simulink subsystem "aeroParamsCalculation"  (R2025b)
settings: Solver=VariableStepAuto  StartTime=0.0  StopTime=10.0  RelTol=1e-3
values from neighbouring files (symbols this model uses):
  aeroParams : value not decoded    [plantParams.sldd]
libraries: simulink_extras x6, matrix_library x4
settings Model: Creator=maxhu  LastModifiedBy=maxhu

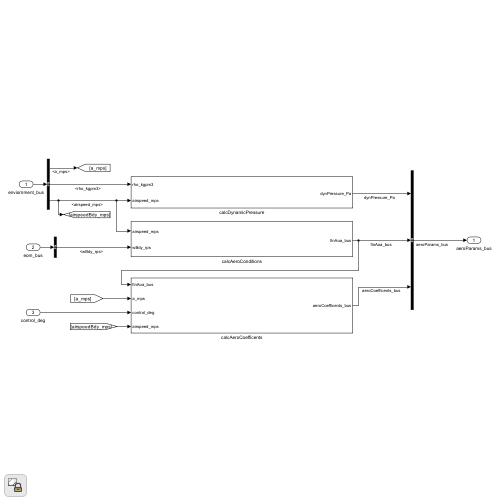
[thumbnail: Simulink's stored preview of the top-level diagram]
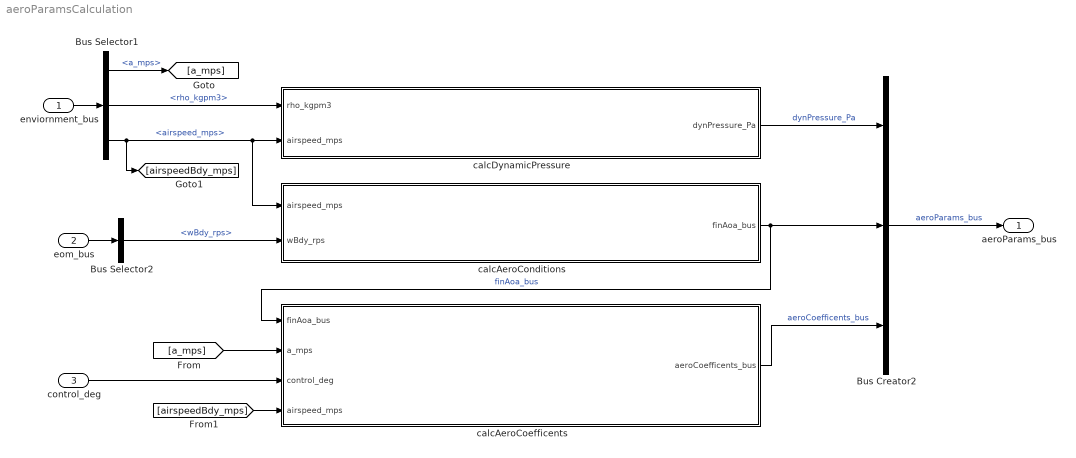
== system aeroParamsCalculation ==
  enviornment_bus : Inport
  eom_bus : Inport  Port=2
  control_deg : Inport  Port=3
  Bus Creator2 : BusCreator  Inputs=3
  Bus Selector1 : BusSelector  OutputSignals=a_mps,rho_kgpm3,airspeed_mps
  Bus Selector2 : BusSelector  OutputSignals=wBdy_rps
  calcAeroCoefficents : Subsystem
  calcAeroConditions : Subsystem
  calcDynamicPressure : Subsystem
  aeroParams_bus : Outport
  wires:
  enviornment_bus/1 -> Bus Selector1/1
  eom_bus/1 -> Bus Selector2/1
  Bus Creator2/1 -> aeroParams_bus/1  "aeroParams_bus"
  Bus Selector2/1 -> calcAeroConditions/2(wBdy_rps)  "<wBdy_rps>"
  Bus Selector1/2 -> calcDynamicPressure/1(rho_kgpm3)  "<rho_kgpm3>"
  calcAeroConditions/1(finAoa_bus) -> calcAeroCoefficents/1(finAoa_bus), Bus Creator2/2  "finAoa_bus"
  calcDynamicPressure/1(dynPressure_Pa) -> Bus Creator2/1  "dynPressure_Pa"
  Bus Selector1/1 -> [a_mps]  "<a_mps>"
  [a_mps] -> calcAeroCoefficents/2(a_mps)
  [airspeedBdy_mps] -> calcAeroCoefficents/4(airspeed_mps)
  control_deg/1 -> calcAeroCoefficents/3(control_deg)
  calcAeroCoefficents/1(aeroCoefficents_bus) -> Bus Creator2/3  "aeroCoefficents_bus"
  Bus Selector1/3 -> calcDynamicPressure/2(airspeed_mps), calcAeroConditions/1(airspeed_mps), [airspeedBdy_mps]  "<airspeed_mps>"

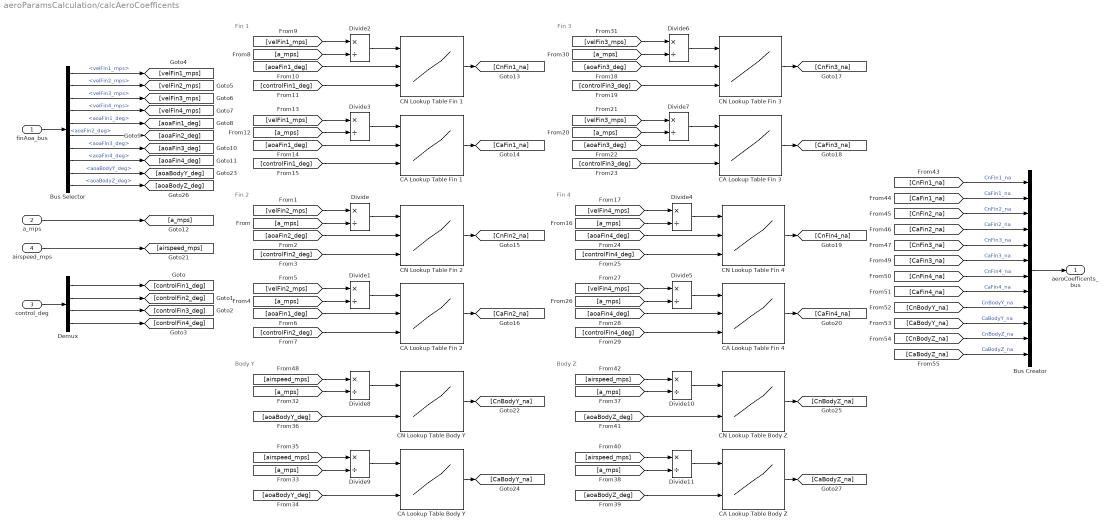
== system aeroParamsCalculation/calcAeroCoefficents ==
  note: Body Y
  note: Body Z
  note: Fin 4
  note: Fin 3
  note: Fin 1
  note: Fin 2
  finAoa_bus : Inport
  a_mps : Inport  Port=2
  control_deg : Inport  Port=3
  airspeed_mps : Inport  Port=4
  Bus Creator : BusCreator  Inputs=12
  Bus Selector : BusSelector  OutputSignals=velFin1_mps,velFin2_mps,velFin3_mps,velFin4_mps,aoaFin1_deg,aoaFin2_deg,aoaFin3_deg,aoaFin4_deg,aoaBodyY_deg,aoaBodyZ_deg
  CA Lookup Table Body Y : Lookup_n-D  BreakpointsForDimension1=aeroParams.machBreakpoints_na  BreakpointsForDimension2=aeroParams.aoaBreakpoints_deg  BreakpointsForDimension3=aeroParams.controlBreakpoints_deg  Table=aeroParams.CaBase_na  InternalRulePriority=Speed  RndMeth=Simplest
      settings: InputPortMap=u0,u1
  CA Lookup Table Body Z : Lookup_n-D  BreakpointsForDimension1=aeroParams.machBreakpoints_na  BreakpointsForDimension2=aeroParams.aoaBreakpoints_deg  BreakpointsForDimension3=aeroParams.controlBreakpoints_deg  Table=aeroParams.CaBase_na  InternalRulePriority=Speed  RndMeth=Simplest
      settings: InputPortMap=u0,u1
  CA Lookup Table Fin {1..4} (4 alike) : Lookup_n-D  NumberOfTableDimensions=3  BreakpointsForDimension1=aeroParams.machBreakpoints_na  BreakpointsForDimension2=aeroParams.aoaBreakpoints_deg  BreakpointsForDimension3=aeroParams.controlBreakpoints_deg  Table=aeroParams.CaFin_na  InternalRulePriority=Speed  RndMeth=Simplest
      settings: InputPortMap=u0,u1,u2
  CN Lookup Table Body Y : Lookup_n-D  BreakpointsForDimension1=aeroParams.machBreakpoints_na  BreakpointsForDimension2=aeroParams.aoaBreakpoints_deg  BreakpointsForDimension3=aeroParams.controlBreakpoints_deg  Table=aeroParams.CnBase_na  InternalRulePriority=Speed  RndMeth=Simplest
      settings: InputPortMap=u0,u1
  CN Lookup Table Body Z : Lookup_n-D  BreakpointsForDimension1=aeroParams.machBreakpoints_na  BreakpointsForDimension2=aeroParams.aoaBreakpoints_deg  BreakpointsForDimension3=aeroParams.controlBreakpoints_deg  Table=aeroParams.CnBase_na  InternalRulePriority=Speed  RndMeth=Simplest
      settings: InputPortMap=u0,u1
  CN Lookup Table Fin {1..4} (4 alike) : Lookup_n-D  NumberOfTableDimensions=3  BreakpointsForDimension1=aeroParams.machBreakpoints_na  BreakpointsForDimension2=aeroParams.aoaBreakpoints_deg  BreakpointsForDimension3=aeroParams.controlBreakpoints_deg  Table=aeroParams.CnFin_na  InternalRulePriority=Speed  RndMeth=Simplest
      settings: InputPortMap=u0,u1,u2
  Demux : Demux
  Divide{,1..11} (12 alike) : Product  Inputs=*/
  aeroCoefficents_bus : Outport
  wires:
  Bus Creator/1 -> aeroCoefficents_bus/1
  [CaBodyZ_na] -> Bus Creator/12  "CaBodyZ_na"
  [CnBodyZ_na] -> Bus Creator/11  "CnBodyZ_na"
  [CaBodyY_na] -> Bus Creator/10  "CaBodyY_na"
  [CnBodyY_na] -> Bus Creator/9  "CnBodyY_na"
  [CaFin4_na] -> Bus Creator/8  "CaFin4_na"
  [CnFin4_na] -> Bus Creator/7  "CnFin4_na"
  [CaFin3_na] -> Bus Creator/6  "CaFin3_na"
  [CnFin3_na] -> Bus Creator/5  "CnFin3_na"
  [CaFin2_na] -> Bus Creator/4  "CaFin2_na"
  [CnFin2_na] -> Bus Creator/3  "CnFin2_na"
  [CaFin1_na] -> Bus Creator/2  "CaFin1_na"
  [CnFin1_na] -> Bus Creator/1  "CnFin1_na"
  [a_mps] -> Divide10/2
  Divide10/1 -> CN Lookup Table Body Z/1
  [aoaBodyZ_deg] -> CN Lookup Table Body Z/2
  CN Lookup Table Body Z/1 -> [CnBodyZ_na]
  [aoaBodyZ_deg] -> CA Lookup Table Body Z/2
  CA Lookup Table Body Z/1 -> [CaBodyZ_na]
  [airspeed_mps] -> Divide11/1
  Divide11/1 -> CA Lookup Table Body Z/1
  [a_mps] -> Divide11/2
  [airspeed_mps] -> Divide10/1
  [airspeed_mps] -> Divide9/1
  [a_mps] -> Divide9/2
  Divide9/1 -> CA Lookup Table Body Y/1
  [aoaBodyY_deg] -> CA Lookup Table Body Y/2
  CA Lookup Table Body Y/1 -> [CaBodyY_na]
  Bus Selector/9 -> [aoaBodyY_deg]  "<aoaBodyY_deg>"
  Bus Selector/10 -> [aoaBodyZ_deg]  "<aoaBodyZ_deg>"
  [airspeed_mps] -> Divide8/1
  [aoaBodyY_deg] -> CN Lookup Table Body Y/2
  CN Lookup Table Body Y/1 -> [CnBodyY_na]
  [a_mps] -> Divide8/2
  Divide8/1 -> CN Lookup Table Body Y/1
  airspeed_mps/1 -> [airspeed_mps]
  CA Lookup Table Fin 4/1 -> [CaFin4_na]
  CN Lookup Table Fin 4/1 -> [CnFin4_na]
  CA Lookup Table Fin 3/1 -> [CaFin3_na]
  CN Lookup Table Fin 3/1 -> [CnFin3_na]
  CN Lookup Table Fin 2/1 -> [CnFin2_na]
  CA Lookup Table Fin 2/1 -> [CaFin2_na]
  CA Lookup Table Fin 1/1 -> [CaFin1_na]
  CN Lookup Table Fin 1/1 -> [CnFin1_na]
  Divide5/1 -> CA Lookup Table Fin 4/1
  [velFin4_mps] -> Divide4/1
  [aoaFin4_deg] -> CN Lookup Table Fin 4/2
  [controlFin4_deg] -> CN Lookup Table Fin 4/3
  [a_mps] -> Divide4/2
  [aoaFin3_deg] -> CN Lookup Table Fin 3/2
  [controlFin4_deg] -> CA Lookup Table Fin 4/3
  Divide6/1 -> CN Lookup Table Fin 3/1
  [aoaFin4_deg] -> CA Lookup Table Fin 4/2
  [a_mps] -> Divide5/2
  [velFin4_mps] -> Divide5/1
  Divide4/1 -> CN Lookup Table Fin 4/1
  [a_mps] -> Divide6/2
  [velFin3_mps] -> Divide7/1
  [aoaFin3_deg] -> CA Lookup Table Fin 3/2
  [controlFin3_deg] -> CA Lookup Table Fin 3/3
  [a_mps] -> Divide7/2
  [controlFin3_deg] -> CN Lookup Table Fin 3/3
  [velFin3_mps] -> Divide6/1
  Divide7/1 -> CA Lookup Table Fin 3/1
  Divide3/1 -> CA Lookup Table Fin 1/1
  [velFin1_mps] -> Divide2/1
  [aoaFin1_deg] -> CN Lookup Table Fin 1/2
  [controlFin1_deg] -> CN Lookup Table Fin 1/3
  [a_mps] -> Divide2/2
  [controlFin1_deg] -> CA Lookup Table Fin 1/3
  [aoaFin1_deg] -> CA Lookup Table Fin 1/2
  [a_mps] -> Divide3/2
  [velFin1_mps] -> Divide3/1
  Divide2/1 -> CN Lookup Table Fin 1/1
  [velFin2_mps] -> Divide1/1
  Divide1/1 -> CA Lookup Table Fin 2/1
  [controlFin2_deg] -> CA Lookup Table Fin 2/3
  [aoaFin1_deg] -> CA Lookup Table Fin 2/2
  [a_mps] -> Divide1/2
  [controlFin2_deg] -> CN Lookup Table Fin 2/3
  Bus Selector/8 -> [aoaFin4_deg]  "<aoaFin4_deg>"
  Bus Selector/7 -> [aoaFin3_deg]  "<aoaFin3_deg>"
  Bus Selector/6 -> [aoaFin2_deg]  "<aoaFin2_deg>"
  Bus Selector/5 -> [aoaFin1_deg]  "<aoaFin1_deg>"
  [aoaFin2_deg] -> CN Lookup Table Fin 2/2
  Divide/1 -> CN Lookup Table Fin 2/1
  [velFin2_mps] -> Divide/1
  [a_mps] -> Divide/2
  a_mps/1 -> [a_mps]
  Bus Selector/4 -> [velFin4_mps]  "<velFin4_mps>"
  Bus Selector/3 -> [velFin3_mps]  "<velFin3_mps>"
  Bus Selector/2 -> [velFin2_mps]  "<velFin2_mps>"
  Bus Selector/1 -> [velFin1_mps]  "<velFin1_mps>"
  finAoa_bus/1 -> Bus Selector/1
  Demux/4 -> [controlFin4_deg]
  Demux/3 -> [controlFin3_deg]
  Demux/2 -> [controlFin2_deg]
  Demux/1 -> [controlFin1_deg]
  control_deg/1 -> Demux/1

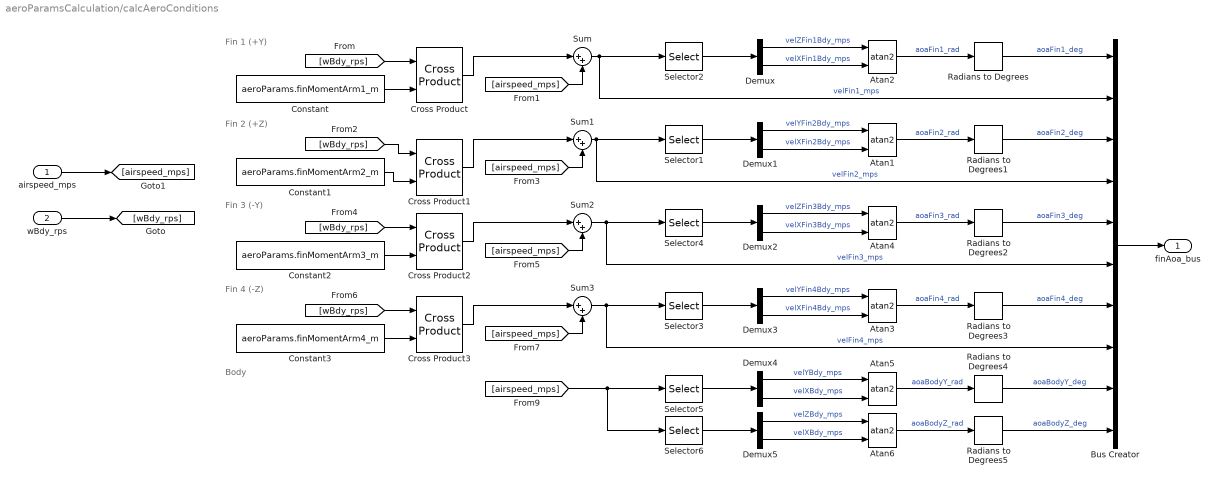
== system aeroParamsCalculation/calcAeroConditions ==
  note: Body
  note: Fin 1 (+Y)
  note: Fin 2 (+Z)
  note: Fin 3 (-Y)
  note: Fin 4 (-Z)
  airspeed_mps : Inport
  wBdy_rps : Inport  Port=2
  Atan{1..6} (6 alike) : Trigonometry  Operator=atan2
  Bus Creator : BusCreator  Inputs=10
  Constant : Constant  Value=aeroParams.finMomentArm1_m
  Constant1 : Constant  Value=aeroParams.finMomentArm2_m
  Constant2 : Constant  Value=aeroParams.finMomentArm3_m
  Constant3 : Constant  Value=aeroParams.finMomentArm4_m
  Cross Product{,1..3} (4 alike) : matrix_library/Cross Product
  Demux{,1..5} (6 alike) : Demux  Outputs=2
  Radians to Degrees{,1..5} (6 alike) : simulink_extras/Transformations/Radians to Degrees
  Selector1 : Selector  InputPortWidth=3  IndexOptions=Index vector (dialog)  Indices=[2 1]  OutputSizes=1
  Selector2 : Selector  InputPortWidth=3  IndexOptions=Index vector (dialog)  Indices=[3 1]  OutputSizes=1
  Selector3 : Selector  InputPortWidth=3  IndexOptions=Index vector (dialog)  Indices=[2 1]  OutputSizes=1
  Selector4 : Selector  InputPortWidth=3  IndexOptions=Index vector (dialog)  Indices=[3 1]  OutputSizes=1
  Selector5 : Selector  InputPortWidth=3  IndexOptions=Index vector (dialog)  Indices=[3 1]  OutputSizes=1
  Selector6 : Selector  InputPortWidth=3  IndexOptions=Index vector (dialog)  Indices=[2 1]  OutputSizes=1
  Sum{,1..3} (4 alike) : Sum  Inputs=|++
  finAoa_bus : Outport
  wires:
  Radians to Degrees5/1 -> Bus Creator/10  "aoaBodyZ_deg"
  Radians to Degrees4/1 -> Bus Creator/9  "aoaBodyY_deg"
  Selector6/1 -> Demux5/1
  Demux5/1 -> Atan6/1  "velZBdy_mps"
  Demux5/2 -> Atan6/2  "velXBdy_mps"
  Atan6/1 -> Radians to Degrees5/1  "aoaBodyZ_rad"
  Selector5/1 -> Demux4/1
  Atan5/1 -> Radians to Degrees4/1  "aoaBodyY_rad"
  Demux4/2 -> Atan5/2  "velXBdy_mps"
  [airspeed_mps] -> Selector6/1, Selector5/1
  Demux4/1 -> Atan5/1  "velYBdy_mps"
  Radians to Degrees3/1 -> Bus Creator/7  "aoaFin4_deg"
  Radians to Degrees2/1 -> Bus Creator/5  "aoaFin3_deg"
  Radians to Degrees1/1 -> Bus Creator/3  "aoaFin2_deg"
  Radians to Degrees/1 -> Bus Creator/1  "aoaFin1_deg"
  Bus Creator/1 -> finAoa_bus/1
  Atan3/1 -> Radians to Degrees3/1  "aoaFin4_rad"
  Atan4/1 -> Radians to Degrees2/1  "aoaFin3_rad"
  Atan1/1 -> Radians to Degrees1/1  "aoaFin2_rad"
  Atan2/1 -> Radians to Degrees/1  "aoaFin1_rad"
  Demux2/1 -> Atan4/1  "velZFin3Bdy_mps"
  Constant2/1 -> Cross Product2/2
  [airspeed_mps] -> Sum2/2
  Selector4/1 -> Demux2/1
  Cross Product2/1 -> Sum2/1
  [wBdy_rps] -> Cross Product2/1
  Sum3/1 -> Selector3/1, Bus Creator/8  "velFin4_mps"
  [wBdy_rps] -> Cross Product3/1
  [airspeed_mps] -> Sum3/2
  Constant3/1 -> Cross Product3/2
  Cross Product3/1 -> Sum3/1
  Selector3/1 -> Demux3/1
  Demux3/1 -> Atan3/1  "velYFin4Bdy_mps"
  Demux3/2 -> Atan3/2  "velXFin4Bdy_mps"
  Demux2/2 -> Atan4/2  "velXFin3Bdy_mps"
  Sum2/1 -> Selector4/1, Bus Creator/6  "velFin3_mps"
  Demux1/1 -> Atan1/1  "velYFin2Bdy_mps"
  Constant1/1 -> Cross Product1/2
  [airspeed_mps] -> Sum1/2
  Selector1/1 -> Demux1/1
  Cross Product1/1 -> Sum1/1
  [wBdy_rps] -> Cross Product1/1
  Demux1/2 -> Atan1/2  "velXFin2Bdy_mps"
  Sum1/1 -> Selector1/1, Bus Creator/4  "velFin2_mps"
  Demux/2 -> Atan2/2  "velXFin1Bdy_mps"
  Demux/1 -> Atan2/1  "velZFin1Bdy_mps"
  Selector2/1 -> Demux/1
  Sum/1 -> Selector2/1, Bus Creator/2  "velFin1_mps"
  [airspeed_mps] -> Sum/2
  Cross Product/1 -> Sum/1
  airspeed_mps/1 -> [airspeed_mps]
  [wBdy_rps] -> Cross Product/1
  Constant/1 -> Cross Product/2
  wBdy_rps/1 -> [wBdy_rps]

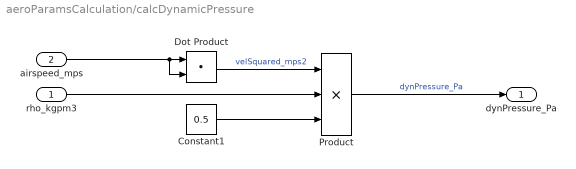
== system aeroParamsCalculation/calcDynamicPressure ==
  rho_kgpm3 : Inport
  airspeed_mps : Inport  Port=2
  Constant1 : Constant  Value=0.5
  Dot Product : DotProduct  OutDataTypeStr=Inherit: Inherit via internal rule
  Product : Product  Inputs=3
  dynPressure_Pa : Outport
  wires:
  rho_kgpm3/1 -> Product/2
  Constant1/1 -> Product/3
  Dot Product/1 -> Product/1  "velSquared_mps2"
  airspeed_mps/1 -> Dot Product/1, Dot Product/2
  Product/1 -> dynPressure_Pa/1  "dynPressure_Pa"
